simulink model "TxSteering_RxMVDR_4x4_HDL_IQ"  (R2023a)
settings: Solver=FixedStepDiscrete  StartTime=0.0  StopTime=stoptime  RelTol=1e-3
PreLoadFcn:
  | model_init
InitFcn:
  | model_init
model workspace (MAT data in the model file):
  socvcb = containers.Map
  socvcb.serialization.keys = {}
  socvcb.serialization.values = {}
  socvcb.serialization.uniformity = 0
  socvcb.serialization.keyType = 'double'
  socvcb.serialization.valueType = 'any'
values from neighbouring files (symbols this model uses):
  diagLoading = 5e-3    (= 0.005)    [model_init.m]
  dmaFIFOLength = 2^nextpow2(testSrc1.FrameLength*testSrc1.SamplesPerSymbol*2)    [model_init.m]
  fc = ConverterSampleRate*7/16    (= 860160000)    [model_init.m]
  FPGAClkRate = DataSampleRate/VectorSamplingFactor    (= 245760000)    [model_init.m]
  movavg_bitshift = nextpow2(windowSize)    [model_init.m]
  mvdrPipelineDelay = covMatDelay+movAvgDelay+matrixSolveDelay+normResponseDelay    [model_init.m]
  NCO_bits = 14    [model_init.m]
  numArrayElements = 4    [model_init.m]
  NumChan = 4    [model_init.m]
  reciprocalDelay = nextpow2(reciprocalin_dt.WordLength) + 1 + reciprocalin_dt.WordLength + 2      - strcmp(reciprocalin_dt.Signedness,'Signed') + 7    [model_init.m]
  rx_mag_delay = input_dt.WordLength + 2 + ceil(log2(NumChan)) + 1 + rx_mag_window_size    [model_init.m]
  rx_mag_inverse_delay = nextpow2(rx_mag_dt.WordLength) + 1 + rx_mag_dt.WordLength + 2 + 7    [model_init.m]
  rx_mag_sum_growth = nextpow2(rx_mag_window_size)    [model_init.m]
  rx_mag_window_size = 256    [model_init.m]
  s2mmFrameSize = testSrc1.FrameLength*testSrc1.SamplesPerSymbol*3    [model_init.m]
  testSrc1 = struct()    [model_init.m]
  testSrc2 = struct()    [model_init.m]
  windowSize = 4096    [model_init.m]
undefined symbols (not defined in the file or in its folder): Add, j, NumBits1, NumBits2, physconst, Shift
libraries: hdlsllib x29, simulink x15, embreciprocals x2, dspsrcs4 x2, dsphdlmathfun2 x1, embsystolicmatrixops x1, dsphdlsigops2 x1, commrfcorlib x1
(part 1 of 3)
Description:
  | MVDR RFSoC example for ZCU111
  | 
  | Copyright 2021 The MathWorks, Inc.
settings Model: DataTypeOverride=Off  SimulationMode=accelerator  Creator=mfornero  LastModifiedBy=tmealey
settings SolverCC: AlgebraicLoopSolver=TrustRegion
settings DataIOCC: SaveOutput=off  SaveTime=off
settings OptimizationCC: BlockReduction=off  ConditionallyExecuteInputs=off  DefaultParameterBehavior=Inlined  ReuseModelBlockBuffer=off  LifeSpan=inf
settings DebuggingCC: AlgebraicLoopMsg=error  SingleTaskRateTransMsg=error  ParameterPrecisionLossMsg=none  UnconnectedInputMsg=warning  UnconnectedOutputMsg=warning  UnconnectedLineMsg=warning  PregeneratedLibrarySubsystemCodeDiagnostic=none  StrictBusMsg=ErrorOnBusTreatedAsVector  SFUnexpectedBacktrackingDiag=warning  SFNoUnconditionalDefaultTransitionDiag=warning  SFExecutionAtInitializationDiag=none  ArithmeticOperatorsInVariantConditions=warning
settings HardwareCC: ProdBitPerPointer=32  ProdBitPerSizeT=32  ProdBitPerPtrDiffT=32  ProdLargestAtomicFloat=None  ProdIntDivRoundTo=Undefined  ProdEndianess=Unspecified  ProdWordSize=32  ProdHWDeviceType=ASIC/FPGA->ASIC/FPGA  ProdEqTarget=off
settings ModelReferenceCC: EnableRefExpFcnMdlSchedulingChecks=on
settings SFSimCC: SimUseLocalCustomCode=off  CustomCodeUndefinedFunction=UseInterfaceOnly
settings RTWCC: RTWUseLocalCustomCode=off  DLArmComputeVersion=19.05
settings CodeAppCC: StateflowObjectComments=on
settings GRTTargetCC: TargetLangStandard=C89/C90 (ANSI)
settings ConfigComp: CovMetricSettings=dw  CovSaveCumulativeToWorkspaceVar=on  CovSaveSingleToWorkspaceVar=on  CovExternalEMLEnable=off

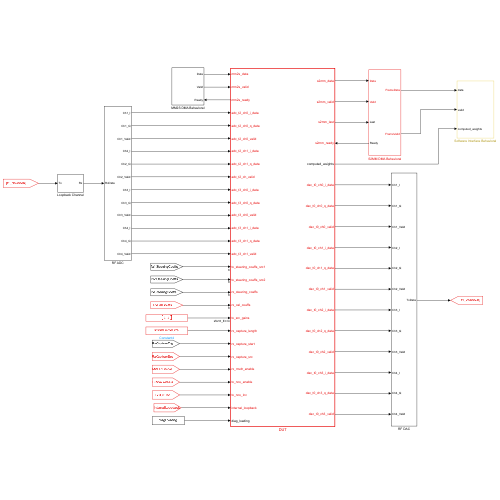
[thumbnail: Simulink's stored preview of the top-level diagram]
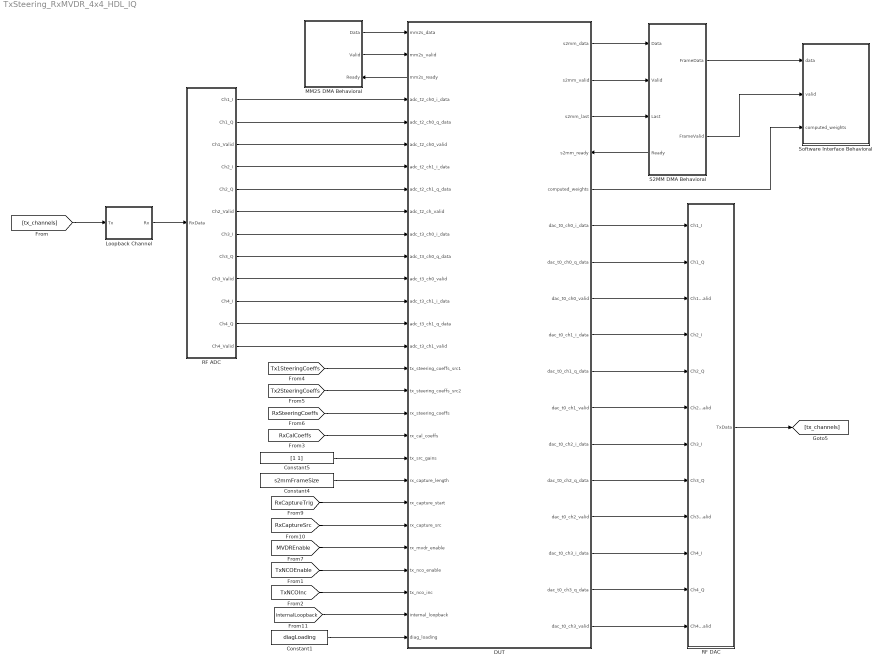
== system TxSteering_RxMVDR_4x4_HDL_IQ ==
  Constant1 : Constant  Value=diagLoading  OutDataTypeStr=matrixdivin_dt  SampleTime=-1
  Constant4 : Constant  Value=s2mmFrameSize  OutDataTypeStr=uint32  SampleTime=-1
  Constant5 : Constant  Value=[1 1]  OutDataTypeStr=tx_gain_dt  SampleTime=-1
  DUT : Subsystem  TreatAsAtomicUnit=on
      settings: PortSchema="{\"entries\":[{\"content\":{\"sides\":[{\"content\":{\"connectorIds\":[\"In1\",\"In2\",\"Out17\",\"In3\",\"In4\",\"In5\",\"In6\",\"In7\",\"In8\",\"In9\",\"In10\",\"In11\",\"In12\",\"In13\",\"In14\",\"In15\",\"In16\",\"In17\",\"In18\",\"In19\",\"In20\",\"In21\",\"In22\",\"In23\",\"In24\",\"In25\",\"In26\",\"In27\"]},\"type\":\"ConnectorPlacement.EquallySpacedRectSide\",\"uuid\":\"5cbbc5c1-13a2-4dd5-b798-0d6aa5a3512c\"},{\"content\":{\"connectorIds\":[\"Out1\",\"Out2\",\"Out3\",\"In28\",\"Out4\",\"Out5\",\"Out6\",\"Out7\",\"Out8\",\"Out9\",\"Out10\",\"Out11\",\"Out12\",\"Out13\",\"Out14\",\"Out15\",\"Out16\"],\"side\":\"RIGHT\"},\"type\":\"ConnectorPlacement.EquallySpacedRectSide\",\"uuid\":\"078c6bc6-159b-4e6a-9020-aaf50b1c87f6\"},{\"content\":{\"side\":\"TOP\"},\"type\":\"ConnectorPlacement.EquallySpacedRectSide\",\"uuid\":\"5dec20bf-c028-4555-acb0-00d4e0bd1eb1\"},{\"content\":{\"side\":\"HIDDEN\"},\"type\":\"ConnectorPlacement.EquallySpacedRectSide\",\"uuid\":\"f104c99f-3c00-46d1-a3ab-da9a095ae20c\"}]},\"type\":\"ConnectorPlacement.EquallySpacedConnector\",\"uuid\":\"99ff154b-6e8c-428f-8f67-53aff3cd9053\"}],\"packageUris\":[\"http://schema.mathworks.com/mf0/Connector/R2020b\"],\"version\":\"1.0\"}"
  Loopback Channel : Subsystem
  MM2S DMA Behavioral : Subsystem
      settings: PortSchema="{\"entries\":[{\"content\":{\"sides\":[{\"content\":{\"connectorIds\":[]},\"type\":\"ConnectorPlacement.EquallySpacedRectSide\",\"uuid\":\"6e5a1ec8-43bd-4e5c-bb67-adc7e52f765e\"},{\"content\":{\"connectorIds\":[\"Out1\",\"Out2\",\"In1\"],\"side\":\"RIGHT\"},\"type\":\"ConnectorPlacement.EquallySpacedRectSide\",\"uuid\":\"3e14b147-97a5-457d-828e-9dc648279d0e\"},{\"content\":{\"connectorIds\":[],\"side\":\"TOP\"},\"type\":\"ConnectorPlacement.EquallySpacedRectSide\",\"uuid\":\"b499ca48-b31e-4779-aede-04dca658d330\"},{\"content\":{\"connectorIds\":[],\"side\":\"HIDDEN\"},\"type\":\"ConnectorPlacement.EquallySpacedRectSide\",\"uuid\":\"e46e2562-9ab1-42db-980c-487b803af873\"}]},\"type\":\"ConnectorPlacement.EquallySpacedConnector\",\"uuid\":\"234057b8-4ead-4b5a-9893-76ff1204f271\"}],\"packageUris\":[\"http://schema.mathworks.com/mf0/Connector/R2020b\"],\"version\":\"1.0\"}"
  RF ADC : Subsystem
  RF DAC : Subsystem
  S2MM DMA Behavioral : Subsystem
      settings: PortSchema="{\"entries\":[{\"content\":{\"sides\":[{\"content\":{\"connectorIds\":[\"In1\",\"In2\",\"In3\",\"Out3\"]},\"type\":\"ConnectorPlacement.EquallySpacedRectSide\",\"uuid\":\"f5aebce5-d24c-432e-8d9d-6ae810fc0a64\"},{\"content\":{\"connectorIds\":[\"Out1\",\"Out2\"],\"side\":\"RIGHT\"},\"type\":\"ConnectorPlacement.EquallySpacedRectSide\",\"uuid\":\"87d7b61c-1b18-489c-87d0-263bc891b967\"},{\"content\":{\"side\":\"TOP\"},\"type\":\"ConnectorPlacement.EquallySpacedRectSide\",\"uuid\":\"c0471b66-642d-47c1-93a8-85d0262e809a\"},{\"content\":{\"side\":\"HIDDEN\"},\"type\":\"ConnectorPlacement.EquallySpacedRectSide\",\"uuid\":\"468d2625-6b9b-4b39-93eb-7f122a4e72a5\"}]},\"type\":\"ConnectorPlacement.EquallySpacedConnector\",\"uuid\":\"6af60fba-ab37-47d2-9d8a-dd48226214e6\"}],\"packageUris\":[\"http://schema.mathworks.com/mf0/Connector/R2020b\"],\"version\":\"1.0\"}"
  Software Interface Behavioral : Subsystem
  wires:
  [InternalLoopback] -> DUT/26(internal_loopback)
  Constant5/1 -> DUT/19(tx_src_gains)
  Constant4/1 -> DUT/20(rx_capture_length)
  [RxCaptureTrig] -> DUT/21(rx_capture_start)
  [RxCaptureSrc] -> DUT/22(rx_capture_src)
  DUT/5(dac_t0_ch0_i_data) -> RF DAC/1(Ch1_I)
  DUT/6(dac_t0_ch0_q_data) -> RF DAC/2(Ch1_Q)
  DUT/7(dac_t0_ch0_valid) -> RF DAC/3(Ch1_Valid)
  DUT/8(dac_t0_ch1_i_data) -> RF DAC/4(Ch2_I)
  DUT/9(dac_t0_ch1_q_data) -> RF DAC/5(Ch2_Q)
  DUT/10(dac_t0_ch1_valid) -> RF DAC/6(Ch2_Valid)
  DUT/11(dac_t0_ch2_i_data) -> RF DAC/7(Ch3_I)
  DUT/12(dac_t0_ch2_q_data) -> RF DAC/8(Ch3_Q)
  DUT/13(dac_t0_ch2_valid) -> RF DAC/9(Ch3_Valid)
  DUT/14(dac_t0_ch3_i_data) -> RF DAC/10(Ch4_I)
  DUT/15(dac_t0_ch3_q_data) -> RF DAC/11(Ch4_Q)
  DUT/16(dac_t0_ch3_valid) -> RF DAC/12(Ch4_Valid)
  RF DAC/1(TxData) -> [tx_channels]
  [tx_channels] -> Loopback Channel/1(Tx)
  Loopback Channel/1(Rx) -> RF ADC/1(RxData)
  [TxNCOEnable] -> DUT/24(tx_nco_enable)
  [TxNCOInc] -> DUT/25(tx_nco_inc)
  S2MM DMA Behavioral/3(Ready) -> DUT/28(s2mm_ready)
  S2MM DMA Behavioral/1(FrameData) -> Software Interface Behavioral/1(data)
  S2MM DMA Behavioral/2(FrameValid) -> Software Interface Behavioral/2(valid)
  DUT/4(computed_weights) -> Software Interface Behavioral/3(computed_weights)
  DUT/1(s2mm_data) -> S2MM DMA Behavioral/1(Data)
  DUT/2(s2mm_valid) -> S2MM DMA Behavioral/2(Valid)
  MM2S DMA Behavioral/1(Data) -> DUT/1(mm2s_data)
  MM2S DMA Behavioral/2(Valid) -> DUT/2(mm2s_valid)
  DUT/17(mm2s_ready) -> MM2S DMA Behavioral/1(Ready)
  RF ADC/6(Ch2_Valid) -> DUT/8(adc_t2_ch_valid)
  RF ADC/7(Ch3_I) -> DUT/9(adc_t3_ch0_i_data)
  RF ADC/8(Ch3_Q) -> DUT/10(adc_t3_ch0_q_data)
  RF ADC/9(Ch3_Valid) -> DUT/11(adc_t3_ch0_valid)
  RF ADC/10(Ch4_I) -> DUT/12(adc_t3_ch1_i_data)
  RF ADC/11(Ch4_Q) -> DUT/13(adc_t3_ch1_q_data)
  RF ADC/12(Ch4_Valid) -> DUT/14(adc_t3_ch1_valid)
  [Tx1SteeringCoeffs] -> DUT/15(tx_steering_coeffs_src1)
  [Tx2SteeringCoeffs] -> DUT/16(tx_steering_coeffs_src2)
  [RxSteeringCoeffs] -> DUT/17(rx_steering_coeffs)
  [RxCalCoeffs] -> DUT/18(rx_cal_coeffs)
  DUT/3(s2mm_last) -> S2MM DMA Behavioral/3(Last)
  [MVDREnable] -> DUT/23(rx_mvdr_enable)
  RF ADC/1(Ch1_I) -> DUT/3(adc_t2_ch0_i_data)
  RF ADC/2(Ch1_Q) -> DUT/4(adc_t2_ch0_q_data)
  RF ADC/3(Ch1_Valid) -> DUT/5(adc_t2_ch0_valid)
  RF ADC/4(Ch2_I) -> DUT/6(adc_t2_ch1_i_data)
  RF ADC/5(Ch2_Q) -> DUT/7(adc_t2_ch1_q_data)
  Constant1/1 -> DUT/27(diag_loading)

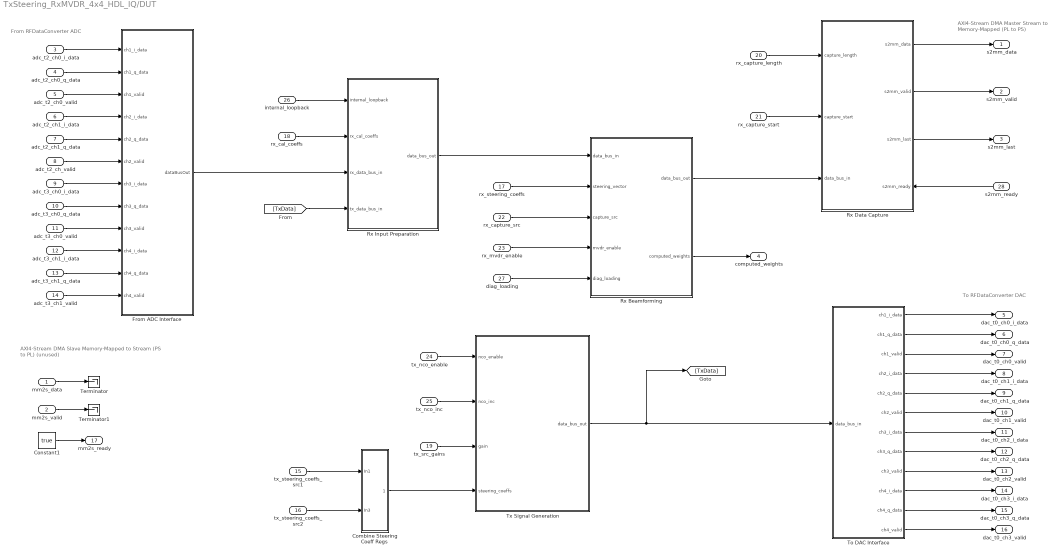
== system TxSteering_RxMVDR_4x4_HDL_IQ/DUT ==
  note: AXI4-Stream DMA Master
      | Stream to Memory-Mapped (PL to PS)
  note: AXI4-Stream DMA Slave
      | Memory-Mapped to Stream (PS to PL)
      | (unused)
  note: From RFDataConverter ADC
  note: To RFDataConverter DAC
  mm2s_data : Inport
  mm2s_valid : Inport  Port=2
  adc_t2_ch0_i_data : Inport  Port=3
  adc_t2_ch0_q_data : Inport  Port=4
  adc_t2_ch0_valid : Inport  Port=5
  adc_t2_ch1_i_data : Inport  Port=6
  adc_t2_ch1_q_data : Inport  Port=7
  adc_t2_ch_valid : Inport  Port=8
  adc_t3_ch0_i_data : Inport  Port=9
  adc_t3_ch0_q_data : Inport  Port=10
  adc_t3_ch0_valid : Inport  Port=11
  adc_t3_ch1_i_data : Inport  Port=12
  adc_t3_ch1_q_data : Inport  Port=13
  adc_t3_ch1_valid : Inport  Port=14
  tx_steering_coeffs_src1 : Inport  Port=15  PortDimensions=NumChan*2
  tx_steering_coeffs_src2 : Inport  Port=16  PortDimensions=NumChan*2
  rx_steering_coeffs : Inport  Port=17  PortDimensions=NumChan*2
  rx_cal_coeffs : Inport  Port=18  PortDimensions=NumChan*2
  tx_src_gains : Inport  Port=19  OutDataTypeStr=tx_gain_dt
  rx_capture_length : Inport  Port=20
  rx_capture_start : Inport  Port=21
  rx_capture_src : Inport  Port=22
  rx_mvdr_enable : Inport  Port=23
  tx_nco_enable : Inport  Port=24
  tx_nco_inc : Inport  Port=25
  internal_loopback : Inport  Port=26
  diag_loading : Inport  Port=27
  s2mm_ready : Inport  Port=28
  Combine Steering Coeff Regs : Subsystem
  Constant1 : Constant  Value=true  OutDataTypeStr=boolean  SampleTime=-1
  From ADC Interface : Subsystem
  Rx Beamforming : Subsystem
  Rx Data Capture : Subsystem
      settings: PortSchema="{\"entries\":[{\"content\":{\"sides\":[{\"content\":{\"connectorIds\":[\"In1\",\"In2\",\"In3\"]},\"type\":\"ConnectorPlacement.EquallySpacedRectSide\",\"uuid\":\"3ce440ad-60a3-40a1-9abc-8b07e8479e74\"},{\"content\":{\"connectorIds\":[\"Out1\",\"Out2\",\"Out3\",\"In4\"],\"side\":\"RIGHT\"},\"type\":\"ConnectorPlacement.EquallySpacedRectSide\",\"uuid\":\"92cb9a6e-31c8-4c68-811d-5cb9de201228\"},{\"content\":{\"side\":\"TOP\"},\"type\":\"ConnectorPlacement.EquallySpacedRectSide\",\"uuid\":\"4ff664a1-3d68-43c3-89c1-825c045b6984\"},{\"content\":{\"side\":\"HIDDEN\"},\"type\":\"ConnectorPlacement.EquallySpacedRectSide\",\"uuid\":\"ea40c324-81e0-4145-89f3-1e0de81d6070\"}]},\"type\":\"ConnectorPlacement.EquallySpacedConnector\",\"uuid\":\"89aac716-5ee7-4b56-a06e-6874cb9890cb\"}],\"packageUris\":[\"http://schema.mathworks.com/mf0/Connector/R2020b\"],\"version\":\"1.0\"}"
  Rx Input Preparation : Subsystem
  Terminator : Terminator
  Terminator1 : Terminator
  To DAC Interface : Subsystem
  Tx Signal Generation : Subsystem
  s2mm_data : Outport  VectorParamsAs1DForOutWhenUnconnected=off
  s2mm_valid : Outport  Port=2  VectorParamsAs1DForOutWhenUnconnected=off
  s2mm_last : Outport  Port=3  VectorParamsAs1DForOutWhenUnconnected=off
  computed_weights : Outport  Port=4
  dac_t0_ch0_i_data : Outport  Port=5  VectorParamsAs1DForOutWhenUnconnected=off
  dac_t0_ch0_q_data : Outport  Port=6  VectorParamsAs1DForOutWhenUnconnected=off
  dac_t0_ch0_valid : Outport  Port=7  VectorParamsAs1DForOutWhenUnconnected=off
  dac_t0_ch1_i_data : Outport  Port=8  VectorParamsAs1DForOutWhenUnconnected=off
  dac_t0_ch1_q_data : Outport  Port=9  VectorParamsAs1DForOutWhenUnconnected=off
  dac_t0_ch1_valid : Outport  Port=10  VectorParamsAs1DForOutWhenUnconnected=off
  dac_t0_ch2_i_data : Outport  Port=11  VectorParamsAs1DForOutWhenUnconnected=off
  dac_t0_ch2_q_data : Outport  Port=12  VectorParamsAs1DForOutWhenUnconnected=off
  dac_t0_ch2_valid : Outport  Port=13  VectorParamsAs1DForOutWhenUnconnected=off
  dac_t0_ch3_i_data : Outport  Port=14  VectorParamsAs1DForOutWhenUnconnected=off
  dac_t0_ch3_q_data : Outport  Port=15  VectorParamsAs1DForOutWhenUnconnected=off
  dac_t0_ch3_valid : Outport  Port=16  VectorParamsAs1DForOutWhenUnconnected=off
  mm2s_ready : Outport  Port=17  VectorParamsAs1DForOutWhenUnconnected=off
  wires:
  Constant1/1 -> mm2s_ready/1
  s2mm_ready/1 -> Rx Data Capture/4(s2mm_ready)
  rx_capture_length/1 -> Rx Data Capture/1(capture_length)
  rx_capture_start/1 -> Rx Data Capture/2(capture_start)
  Rx Data Capture/2(s2mm_valid) -> s2mm_valid/1
  Rx Data Capture/1(s2mm_data) -> s2mm_data/1
  adc_t2_ch0_i_data/1 -> From ADC Interface/1("ch1_i_data ")
  adc_t2_ch0_valid/1 -> From ADC Interface/3(ch1_valid)
  adc_t2_ch0_q_data/1 -> From ADC Interface/2(ch1_q_data)
  adc_t2_ch1_i_data/1 -> From ADC Interface/4(ch2_i_data)
  adc_t2_ch_valid/1 -> From ADC Interface/6(ch2_valid)
  adc_t2_ch1_q_data/1 -> From ADC Interface/5(ch2_q_data)
  adc_t3_ch0_i_data/1 -> From ADC Interface/7(ch3_i_data)
  adc_t3_ch0_valid/1 -> From ADC Interface/9(ch3_valid)
  adc_t3_ch0_q_data/1 -> From ADC Interface/8(ch3_q_data)
  adc_t3_ch1_i_data/1 -> From ADC Interface/10(ch4_i_data)
  adc_t3_ch1_valid/1 -> From ADC Interface/12(ch4_valid)
  adc_t3_ch1_q_data/1 -> From ADC Interface/11(ch4_q_data)
  mm2s_data/1 -> Terminator/1
  mm2s_valid/1 -> Terminator1/1
  To DAC Interface/1(ch1_i_data) -> dac_t0_ch0_i_data/1
  To DAC Interface/2(ch1_q_data) -> dac_t0_ch0_q_data/1
  To DAC Interface/3(ch1_valid) -> dac_t0_ch0_valid/1
  To DAC Interface/4(ch2_i_data) -> dac_t0_ch1_i_data/1
  To DAC Interface/5(ch2_q_data) -> dac_t0_ch1_q_data/1
  To DAC Interface/6(ch2_valid) -> dac_t0_ch1_valid/1
  To DAC Interface/7(ch3_i_data) -> dac_t0_ch2_i_data/1
  To DAC Interface/8(ch3_q_data) -> dac_t0_ch2_q_data/1
  To DAC Interface/9(ch3_valid) -> dac_t0_ch2_valid/1
  To DAC Interface/10(ch4_i_data) -> dac_t0_ch3_i_data/1
  To DAC Interface/11(ch4_q_data) -> dac_t0_ch3_q_data/1
  To DAC Interface/12(ch4_valid) -> dac_t0_ch3_valid/1
  rx_steering_coeffs/1 -> Rx Beamforming/2(steering_vector)
  tx_steering_coeffs_src1/1 -> Combine Steering Coeff Regs/1(In1)
  tx_steering_coeffs_src2/1 -> Combine Steering Coeff Regs/2(In3)
  [TxData] -> Rx Input Preparation/4(tx_data_bus_in)
  rx_capture_src/1 -> Rx Beamforming/3(capture_src)
  internal_loopback/1 -> Rx Input Preparation/1(internal_loopback)
  rx_cal_coeffs/1 -> Rx Input Preparation/2(rx_cal_coeffs)
  Tx Signal Generation/1(data_bus_out) -> [TxData], To DAC Interface/1(data_bus_in)
  Combine Steering Coeff Regs/1(Out1) -> Tx Signal Generation/4(steering_coeffs)
  tx_src_gains/1 -> Tx Signal Generation/3(gain)
  Rx Input Preparation/1(data_bus_out) -> Rx Beamforming/1(data_bus_in)
  From ADC Interface/1(dataBusOut) -> Rx Input Preparation/3(rx_data_bus_in)
  tx_nco_inc/1 -> Tx Signal Generation/2(nco_inc)
  tx_nco_enable/1 -> Tx Signal Generation/1(nco_enable)
  Rx Beamforming/2(computed_weights) -> computed_weights/1
  Rx Beamforming/1(data_bus_out) -> Rx Data Capture/3(data_bus_in)
  Rx Data Capture/3(s2mm_last) -> s2mm_last/1
  rx_mvdr_enable/1 -> Rx Beamforming/4(mvdr_enable)
  diag_loading/1 -> Rx Beamforming/5(diag_loading)

== system TxSteering_RxMVDR_4x4_HDL_IQ/Loopback Channel ==
  Tx : Inport
  Apply Channel Noise : Subsystem
  Apply Phase/Amplitude imbalance : Subsystem
  Delay1 : Delay  DelayLength=1
  Gain : Gain  Gain=0.15
  Rx : Outport
  wires:
  Tx/1 -> Delay1/1
  Delay1/1 -> Gain/1
  Apply Phase/Amplitude imbalance/1(Out1) -> Apply Channel Noise/1(In1)
  Apply Channel Noise/1(Rx) -> Rx/1
  Gain/1 -> Apply Phase/Amplitude imbalance/1(In1)

== system TxSteering_RxMVDR_4x4_HDL_IQ/MM2S DMA Behavioral ==
  Ready : Inport
  Constant6 : Constant  Value=false  SampleTime=-1
  Constant7 : Constant  Value=0  OutDataTypeStr=fixdt(0,128,0)  SampleTime=-1
  Terminator : Terminator
  Data : Outport
  Valid : Outport  Port=2
  wires:
  Constant7/1 -> Data/1
  Constant6/1 -> Valid/1
  Ready/1 -> Terminator/1

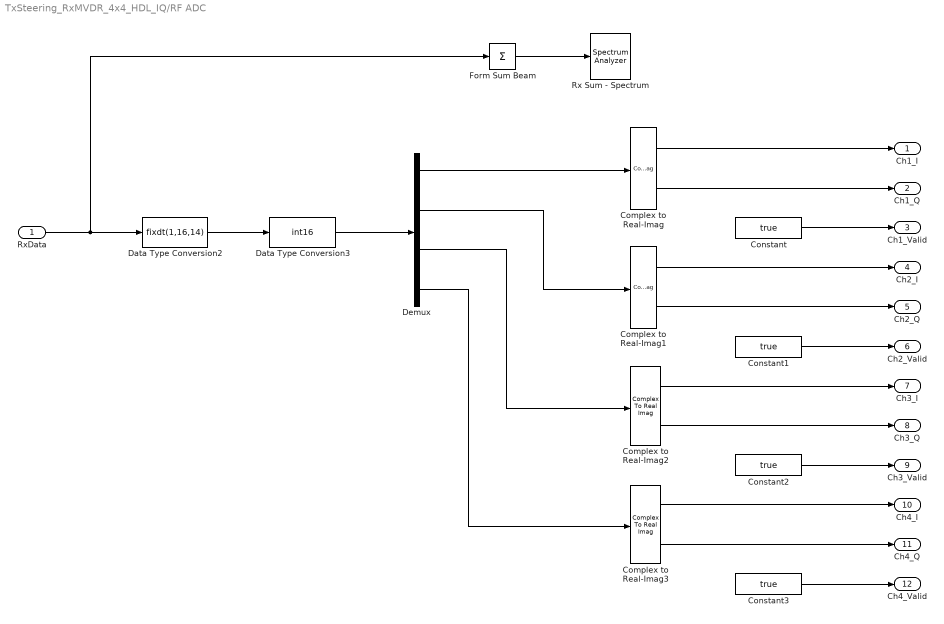
== system TxSteering_RxMVDR_4x4_HDL_IQ/RF ADC ==
  RxData : Inport
  Complex to Real-Imag{,1..3} (4 alike) : ComplexToRealImag
  Constant{,1..3} (4 alike) : Constant  Value=true  SampleTime=-1
  Data Type Conversion2 : DataTypeConversion  OutDataTypeStr=fixdt(1,16,14)  SaturateOnIntegerOverflow=off  RndMeth=Floor
  Data Type Conversion3 : DataTypeConversion  OutDataTypeStr=int16  ConvertRealWorld=Stored Integer (SI)  SaturateOnIntegerOverflow=off  RndMeth=Floor
  Demux : Demux
  Form Sum Beam : Sum  Inputs=+
  Rx Sum - Spectrum : SpectrumAnalyzer  WindowPosition=[121.000000,133.000000,676.000000,509.000000,]  ScopeFrameLocation=window  Method=Welch  SampleRateSource=Property  SampleRate=DataSampleRate  Span=245760000  StartFrequency=-122880000  StopFrequency=122880000  AveragingMethod=Running  YLimits=[-95.95739742,7.93018941]
      settings: OpenAtSimulationStart=off
  Ch1_I : Outport
  Ch1_Q : Outport  Port=2
  Ch1_Valid : Outport  Port=3
  Ch2_I : Outport  Port=4
  Ch2_Q : Outport  Port=5
  Ch2_Valid : Outport  Port=6
  Ch3_I : Outport  Port=7
  Ch3_Q : Outport  Port=8
  Ch3_Valid : Outport  Port=9
  Ch4_I : Outport  Port=10
  Ch4_Q : Outport  Port=11
  Ch4_Valid : Outport  Port=12
  wires:
  Demux/4 -> Complex to Real-Imag3/1
  Complex to Real-Imag1/1 -> Ch2_I/1
  Demux/2 -> Complex to Real-Imag1/1
  Complex to Real-Imag2/2 -> Ch3_Q/1
  Complex to Real-Imag3/1 -> Ch4_I/1
  Demux/3 -> Complex to Real-Imag2/1
  Complex to Real-Imag2/1 -> Ch3_I/1
  Complex to Real-Imag3/2 -> Ch4_Q/1
  Complex to Real-Imag/2 -> Ch1_Q/1
  Complex to Real-Imag/1 -> Ch1_I/1
  Complex to Real-Imag1/2 -> Ch2_Q/1
  Constant/1 -> Ch1_Valid/1
  Demux/1 -> Complex to Real-Imag/1
  Constant1/1 -> Ch2_Valid/1
  Constant2/1 -> Ch3_Valid/1
  Constant3/1 -> Ch4_Valid/1
  Form Sum Beam/1 -> Rx Sum - Spectrum/1
  Data Type Conversion2/1 -> Data Type Conversion3/1
  Data Type Conversion3/1 -> Demux/1
  RxData/1 -> Form Sum Beam/1, Data Type Conversion2/1

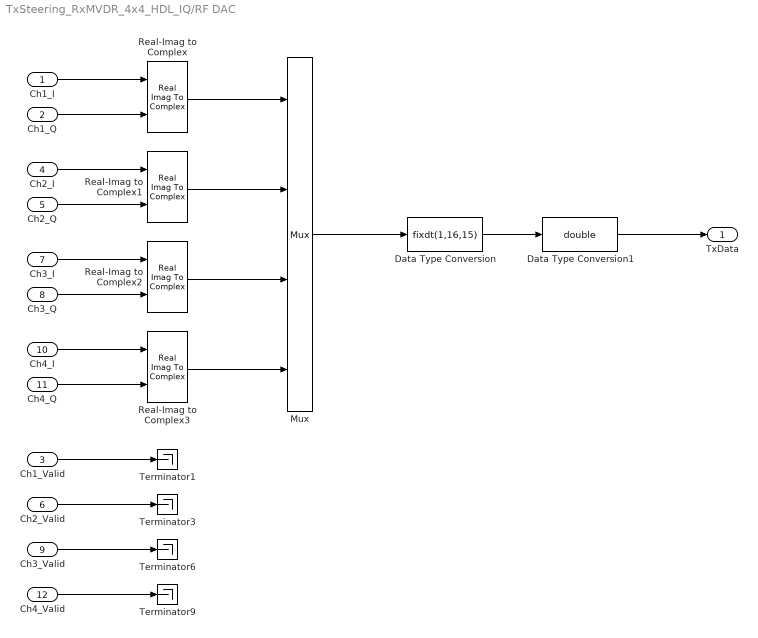
== system TxSteering_RxMVDR_4x4_HDL_IQ/RF DAC ==
  Ch1_I : Inport
  Ch1_Q : Inport  Port=2
  Ch1_Valid : Inport  Port=3
  Ch2_I : Inport  Port=4
  Ch2_Q : Inport  Port=5
  Ch2_Valid : Inport  Port=6
  Ch3_I : Inport  Port=7
  Ch3_Q : Inport  Port=8
  Ch3_Valid : Inport  Port=9
  Ch4_I : Inport  Port=10
  Ch4_Q : Inport  Port=11
  Ch4_Valid : Inport  Port=12
  Data Type Conversion : DataTypeConversion  OutDataTypeStr=fixdt(1,16,15)  ConvertRealWorld=Stored Integer (SI)  SaturateOnIntegerOverflow=off  RndMeth=Floor
  Data Type Conversion1 : DataTypeConversion  OutDataTypeStr=double  SaturateOnIntegerOverflow=off  RndMeth=Floor
  Mux : Mux
  Real-Imag to Complex{,1..3} (4 alike) : RealImagToComplex
  Terminator{1,3,6,9} (4 alike) : Terminator
  TxData : Outport
  wires:
  Ch2_Q/1 -> Real-Imag to Complex1/2
  Ch2_Valid/1 -> Terminator3/1
  Ch3_Valid/1 -> Terminator6/1
  Ch1_Valid/1 -> Terminator1/1
  Ch4_I/1 -> Real-Imag to Complex3/1
  Ch4_Q/1 -> Real-Imag to Complex3/2
  Ch3_Q/1 -> Real-Imag to Complex2/2
  Ch4_Valid/1 -> Terminator9/1
  Ch1_Q/1 -> Real-Imag to Complex/2
  Ch1_I/1 -> Real-Imag to Complex/1
  Ch2_I/1 -> Real-Imag to Complex1/1
  Ch3_I/1 -> Real-Imag to Complex2/1
  Real-Imag to Complex/1 -> Mux/1
  Real-Imag to Complex1/1 -> Mux/2
  Real-Imag to Complex2/1 -> Mux/3
  Real-Imag to Complex3/1 -> Mux/4
  Data Type Conversion/1 -> Data Type Conversion1/1
  Mux/1 -> Data Type Conversion/1
  Data Type Conversion1/1 -> TxData/1

== system TxSteering_RxMVDR_4x4_HDL_IQ/S2MM DMA Behavioral ==
  Data : Inport
  Valid : Inport  Port=2
  Last : Inport  Port=3
  AXI Stream Deserializer : MATLAB Function  TreatAsAtomicUnit=on  mask{FRAME_SIZE=s2mmFrameSize}
      mask prompts: FRAME_SIZE "Frame size:"
  Constant10 : Constant  Value=true  SampleTime=-1
  Delay : Delay  DelayLength=1
  Delay1 : Delay  DelayLength=1
  To Workspace : ToWorkspace  VariableName=sim_dma_valid  SampleTime=-1
      settings: Save2DSignal=2-D array (concatenate along first dimension)
  To Workspace1 : ToWorkspace  VariableName=sim_dma_last  SampleTime=-1
      settings: Save2DSignal=2-D array (concatenate along first dimension)
  To Workspace2 : ToWorkspace  VariableName=sim_dma_data  SampleTime=-1
      settings: Save2DSignal=2-D array (concatenate along first dimension)
  Unpack to uint32 : Subsystem
  FrameData : Outport
  FrameValid : Outport  Port=2
  Ready : Outport  Port=3
  wires:
  Data/1 -> To Workspace2/1, AXI Stream Deserializer/1(data_i)
  Valid/1 -> To Workspace/1, AXI Stream Deserializer/2(valid_i)
  Constant10/1 -> Ready/1
  AXI Stream Deserializer/1(data_o) -> Delay/1
  AXI Stream Deserializer/2(valid_o) -> Delay1/1
  Unpack to uint32/1(dataOut) -> FrameData/1
  Unpack to uint32/2(validOut) -> FrameValid/1
  Delay/1 -> Unpack to uint32/1(dataIn)
  Delay1/1 -> Unpack to uint32/2(validIn)
  Last/1 -> To Workspace1/1

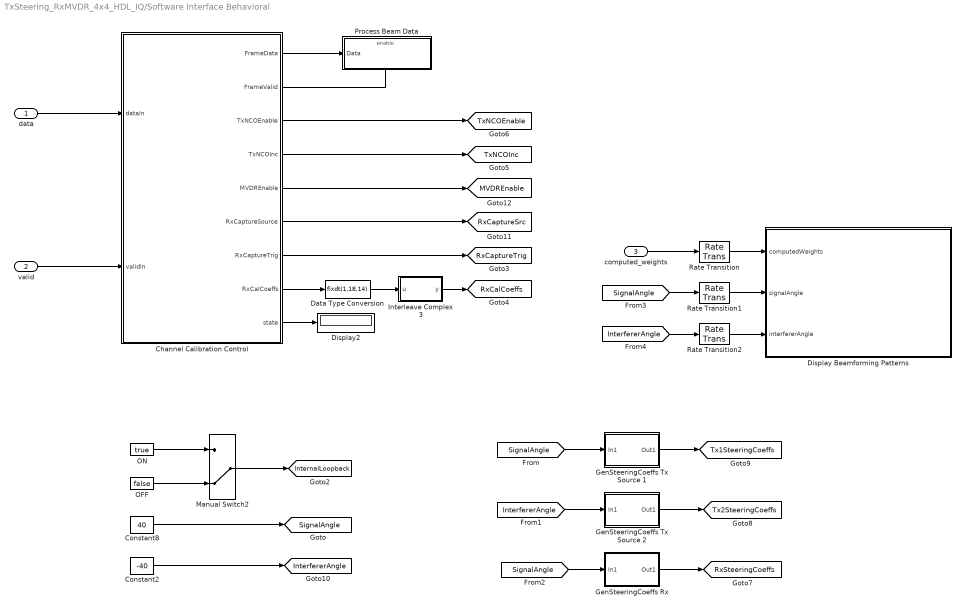
== system TxSteering_RxMVDR_4x4_HDL_IQ/Software Interface Behavioral ==
  data : Inport
  valid : Inport  Port=2
  computed_weights : Inport  Port=3
  Channel Calibration Control : MATLAB Function  TreatAsAtomicUnit=on
      mask init:
      | % Suppress warning for overflow from reinterpretcast
      | Simulink.suppressDiagnostic(gcb,...
      |  'Stateflow:Runtime:DataOverflowErrorMSLD');
  Constant2 : Constant  Value=-40  OutDataTypeStr=double  SampleTime=-1
  Constant8 : Constant  Value=40  OutDataTypeStr=double  SampleTime=-1
  Data Type Conversion : DataTypeConversion  OutDataTypeStr=fixdt(1,18,14)  SaturateOnIntegerOverflow=off  RndMeth=Floor
  Display Beamforming Patterns : MATLAB Function  TreatAsAtomicUnit=on
  Display2 : Display
  GenSteeringCoeffs Rx : Subsystem
  GenSteeringCoeffs Tx Source 1 : Subsystem
  GenSteeringCoeffs Tx Source 2 : Subsystem
  Interleave Complex 3 : Subsystem  mask(Interleave Complex){}
      mask help: Interleave real and imaginary components. Output is a vector with twice the length of the input.
      mask Display: fprintf('Interleave\nComplex');
  Manual Switch2 : ManualSwitch  CurrentSetting=0
  OFF : Constant  Value=false  OutDataTypeStr=boolean  SampleTime=-1
  ON : Constant  Value=true  OutDataTypeStr=boolean  SampleTime=-1
  Process Beam Data : Subsystem
  Rate Transition : RateTransition  OutPortSampleTimeOpt=Multiple of input port sample time  OutPortSampleTimeMultiple=256
  Rate Transition1 : RateTransition  OutPortSampleTimeOpt=Multiple of input port sample time  OutPortSampleTimeMultiple=256
  Rate Transition2 : RateTransition  OutPortSampleTimeOpt=Multiple of input port sample time  OutPortSampleTimeMultiple=256
  tag scope: InterfererAngle=global, InternalLoopback=global, MVDREnable=global, RxCalCoeffs=global, RxCaptureSrc=global, RxCaptureTrig=global, RxSteeringCoeffs=global, SignalAngle=global, Tx1SteeringCoeffs=global, Tx2SteeringCoeffs=global, TxNCOEnable=global, TxNCOInc=global
  wires:
  Channel Calibration Control/5(MVDREnable) -> [MVDREnable]
  OFF/1 -> Manual Switch2/2
  Manual Switch2/1 -> [InternalLoopback]
  ON/1 -> Manual Switch2/1
  data/1 -> Channel Calibration Control/1(dataIn)
  valid/1 -> Channel Calibration Control/2(validIn)
  Channel Calibration Control/4(TxNCOInc) -> [TxNCOInc]
  Channel Calibration Control/3(TxNCOEnable) -> [TxNCOEnable]
  Channel Calibration Control/1(FrameData) -> Process Beam Data/1(Data)
  GenSteeringCoeffs Rx/1(Out1) -> [RxSteeringCoeffs]
  GenSteeringCoeffs Tx Source 2/1(Out1) -> [Tx2SteeringCoeffs]
  GenSteeringCoeffs Tx Source 1/1(Out1) -> [Tx1SteeringCoeffs]
  Constant8/1 -> [SignalAngle]
  Constant2/1 -> [InterfererAngle]
  [SignalAngle] -> GenSteeringCoeffs Tx Source 1/1(In1)
  [InterfererAngle] -> GenSteeringCoeffs Tx Source 2/1(In1)
  [SignalAngle] -> GenSteeringCoeffs Rx/1(In1)
  computed_weights/1 -> Rate Transition/1
  [SignalAngle] -> Rate Transition1/1
  [InterfererAngle] -> Rate Transition2/1
  Rate Transition/1 -> Display Beamforming Patterns/1(computedWeights)
  Rate Transition1/1 -> Display Beamforming Patterns/2(signalAngle)
  Rate Transition2/1 -> Display Beamforming Patterns/3(interfererAngle)
  Channel Calibration Control/2(FrameValid) -> Process Beam Data/Enable
  Data Type Conversion/1 -> Interleave Complex 3/1(u)
  Channel Calibration Control/8(RxCalCoeffs) -> Data Type Conversion/1
  Interleave Complex 3/1(y) -> [RxCalCoeffs]
  Channel Calibration Control/6(RxCaptureSource) -> [RxCaptureSrc]
  Channel Calibration Control/7(RxCaptureTrig) -> [RxCaptureTrig]
  Channel Calibration Control/9(state) -> Display2/1

== system TxSteering_RxMVDR_4x4_HDL_IQ/DUT/Combine Steering Coeff Regs ==
  In1 : Inport
  In3 : Inport  Port=2
  Deinterleave Complex : Subsystem  mask(Deinterleave Complex){}
      mask help: Deinterleave real and imaginary components from input vector. Output is a vector with half the length of the input.
      mask Display: fprintf('Deinterleave\nComplex');
  Deinterleave Complex1 : Subsystem  mask(Deinterleave Complex){}
      mask help: Deinterleave real and imaginary components from input vector. Output is a vector with half the length of the input.
      mask Display: fprintf('Deinterleave\nComplex');
  Vector Concatenate : Concatenate
  Out1 : Outport
  wires:
  Vector Concatenate/1 -> Out1/1
  Deinterleave Complex/1(y) -> Vector Concatenate/1
  In1/1 -> Deinterleave Complex/1(u)
  In3/1 -> Deinterleave Complex1/1(u)
  Deinterleave Complex1/1(y) -> Vector Concatenate/2

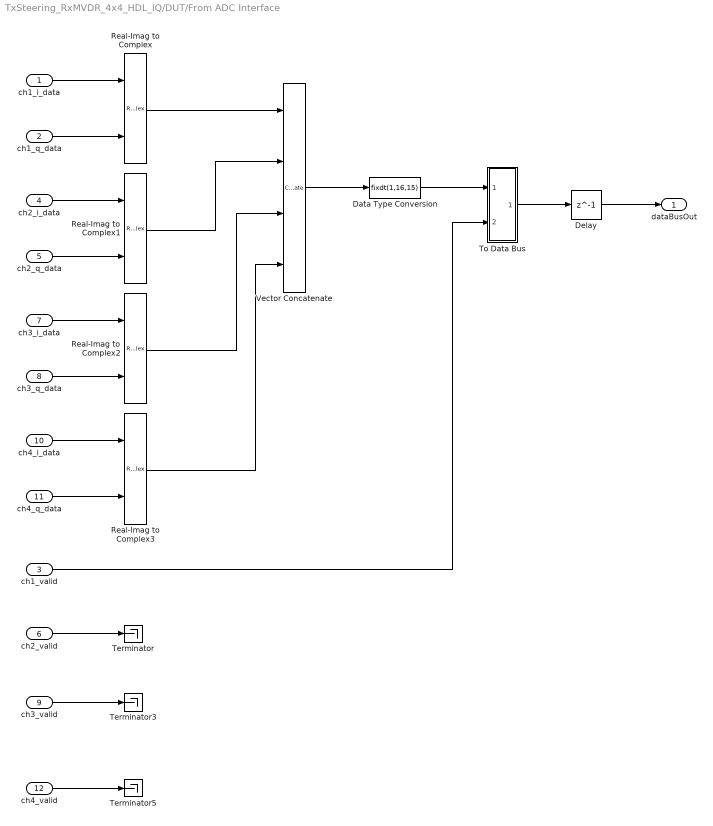
== system TxSteering_RxMVDR_4x4_HDL_IQ/DUT/From ADC Interface ==
  "ch1_i_data " : Inport
  ch1_q_data : Inport  Port=2
  ch1_valid : Inport  Port=3
  ch2_i_data : Inport  Port=4
  ch2_q_data : Inport  Port=5
  ch2_valid : Inport  Port=6
  ch3_i_data : Inport  Port=7
  ch3_q_data : Inport  Port=8
  ch3_valid : Inport  Port=9
  ch4_i_data : Inport  Port=10
  ch4_q_data : Inport  Port=11
  ch4_valid : Inport  Port=12
  Data Type Conversion : DataTypeConversion  OutDataTypeStr=fixdt(1,16,15)  ConvertRealWorld=Stored Integer (SI)  SaturateOnIntegerOverflow=off  RndMeth=Floor
  Delay : Delay  DelayLength=1
  Real-Imag to Complex{,1..3} (4 alike) : RealImagToComplex
  Terminator : Terminator
  Terminator3 : Terminator
  Terminator5 : Terminator
  To Data Bus : Subsystem  mask(To Data Bus){dummy=0}
      mask help: Create a streaming Data Bus from Data and Valid signals.
      mask Display:
      | port_label('input',1,'data');
      | port_label('input',2,'valid');
  Vector Concatenate : Concatenate  NumInputs=4  Mode=Multidimensional array  ConcatenateDimension=2
  dataBusOut : Outport  VectorParamsAs1DForOutWhenUnconnected=off
  wires:
  ch2_valid/1 -> Terminator/1
  ch3_valid/1 -> Terminator3/1
  ch4_valid/1 -> Terminator5/1
  Real-Imag to Complex/1 -> Vector Concatenate/1
  Real-Imag to Complex1/1 -> Vector Concatenate/2
  Real-Imag to Complex2/1 -> Vector Concatenate/3
  Real-Imag to Complex3/1 -> Vector Concatenate/4
  "ch1_i_data "/1 -> Real-Imag to Complex/1
  ch1_q_data/1 -> Real-Imag to Complex/2
  ch2_i_data/1 -> Real-Imag to Complex1/1
  ch2_q_data/1 -> Real-Imag to Complex1/2
  ch3_i_data/1 -> Real-Imag to Complex2/1
  ch3_q_data/1 -> Real-Imag to Complex2/2
  ch4_i_data/1 -> Real-Imag to Complex3/1
  ch4_q_data/1 -> Real-Imag to Complex3/2
  Vector Concatenate/1 -> Data Type Conversion/1
  ch1_valid/1 -> To Data Bus/2(valid)
  To Data Bus/1(bus) -> Delay/1
  Data Type Conversion/1 -> To Data Bus/1(data)
  Delay/1 -> dataBusOut/1

== system TxSteering_RxMVDR_4x4_HDL_IQ/DUT/Rx Beamforming ==
  data_bus_in : Inport
  steering_vector : Inport  Port=2
  capture_src : Inport  Port=3
  mvdr_enable : Inport  Port=4
  diag_loading : Inport  Port=5
  Deinterleave Complex : Subsystem  mask(Deinterleave Complex){}
      mask help: Deinterleave real and imaginary components from input vector. Output is a vector with half the length of the input.
      mask Display: fprintf('Deinterleave\nComplex');
  Input Gate : Subsystem
  Input Scaling : Subsystem
  "Interleave Complex " : Subsystem  mask(Interleave Complex){}
      mask help: Interleave real and imaginary components. Output is a vector with twice the length of the input.
      mask Display: fprintf('Interleave\nComplex');
  MVDR HDL : Subsystem
  Output Selector : Subsystem
  data_bus_out : Outport
  computed_weights : Outport  Port=2
  wires:
  Output Selector/1(data_bus_out) -> data_bus_out/1
  steering_vector/1 -> Deinterleave Complex/1(u)
  MVDR HDL/1(data_bus_out) -> Output Selector/4(mvdr_out_bus)
  data_bus_in/1 -> Output Selector/2(adc_data_bus), Input Scaling/1(data_bus_in)
  MVDR HDL/2(computed_weights) -> "Interleave Complex "/1(u)
  "Interleave Complex "/1(y) -> computed_weights/1
  Deinterleave Complex/1(y) -> MVDR HDL/2(steering_vector)
  mvdr_enable/1 -> Input Gate/1(enable)
  capture_src/1 -> Output Selector/1(src_sel)
  Input Scaling/1(data_bus_out) -> Input Gate/2(data_bus_in)
  Input Gate/1(mvdr_in_bus) -> Output Selector/3(mvdr_in_bus), MVDR HDL/1(data_bus_in)
  diag_loading/1 -> MVDR HDL/3(diag_loading)

== system TxSteering_RxMVDR_4x4_HDL_IQ/DUT/Rx Data Capture ==
  capture_length : Inport
  capture_start : Inport  Port=2
  Bus Element In : Inport  Port=3  PortName=data_bus_in  Element=data
  Bus Element In1 : Inport  Port=3  PortName=data_bus_in  Element=valid
  s2mm_ready : Inport  Port=4
  Delay{,1..2,4} (4 alike) : Delay  DelayLength=1
  Detect Rise Positive : simulink/Logic and Bit Operations/Detect Rise Positive  vinit=0  OutDataTypeStr=boolean
  One-Shot Capture Control : Subsystem
      settings: PortSchema="{\"entries\":[{\"content\":{\"sides\":[{\"content\":{\"connectorIds\":[\"In1\",\"In2\",\"In3\"]},\"type\":\"ConnectorPlacement.EquallySpacedRectSide\",\"uuid\":\"6f09e145-48ee-41d2-bec3-6a733c9106b2\"},{\"content\":{\"connectorIds\":[\"Out1\",\"Out2\",\"In4\"],\"side\":\"RIGHT\"},\"type\":\"ConnectorPlacement.EquallySpacedRectSide\",\"uuid\":\"546a5f38-a809-4883-a76f-61cab94f6d84\"},{\"content\":{\"side\":\"TOP\"},\"type\":\"ConnectorPlacement.EquallySpacedRectSide\",\"uuid\":\"11739b25-d16f-46c4-9eb7-ceb525177655\"}]},\"type\":\"ConnectorPlacement.EquallySpacedConnector\",\"uuid\":\"2379cc98-1392-4372-a564-c1eaf6dbd020\"}],\"packageUris\":[\"http://schema.mathworks.com/mf0/Connector/R2020b\"],\"version\":\"1.0\"}"
  Stream FIFO : Subsystem
      settings: PortSchema="{\"entries\":[{\"content\":{\"sides\":[{\"content\":{\"connectorIds\":[\"In1\",\"In2\",\"In3\",\"Out4\"]},\"type\":\"ConnectorPlacement.EquallySpacedRectSide\",\"uuid\":\"d06c0eab-b8f3-426a-85c0-c3dabc96b0eb\"},{\"content\":{\"connectorIds\":[\"Out1\",\"Out2\",\"Out3\",\"In4\"],\"side\":\"RIGHT\"},\"type\":\"ConnectorPlacement.EquallySpacedRectSide\",\"uuid\":\"fc299245-065a-4284-92f2-e933e11c4572\"},{\"content\":{\"side\":\"TOP\"},\"type\":\"ConnectorPlacement.EquallySpacedRectSide\",\"uuid\":\"8e810d87-ed8e-4951-8437-f6335fefacf7\"}]},\"type\":\"ConnectorPlacement.EquallySpacedConnector\",\"uuid\":\"c15e4701-36e6-4d1a-8e5e-6e8c97e61f22\"}],\"packageUris\":[\"http://schema.mathworks.com/mf0/Connector/R2020b\"],\"version\":\"1.0\"}"
  s2mm_data : Outport  VectorParamsAs1DForOutWhenUnconnected=off
  s2mm_valid : Outport  Port=2  VectorParamsAs1DForOutWhenUnconnected=off
  s2mm_last : Outport  Port=3  VectorParamsAs1DForOutWhenUnconnected=off
  wires:
  capture_length/1 -> Delay2/1
  Bus Element In1/1 -> Delay1/1
  Bus Element In/1 -> Delay/1
  capture_start/1 -> Delay4/1
  Stream FIFO/4(readyOut) -> One-Shot Capture Control/4(readyIn)
  Delay1/1 -> One-Shot Capture Control/1(validIn)
  Delay2/1 -> One-Shot Capture Control/3(length)
  Delay4/1 -> Detect Rise Positive/1
  Detect Rise Positive/1 -> One-Shot Capture Control/2(start)
  Delay/1 -> Stream FIFO/1(dataIn)
  One-Shot Capture Control/1(validOut) -> Stream FIFO/2(validIn)
  Stream FIFO/1(dataOut) -> s2mm_data/1
  Stream FIFO/2(validOut) -> s2mm_valid/1
  s2mm_ready/1 -> Stream FIFO/4(readyIn)
  One-Shot Capture Control/2(lastOut) -> Stream FIFO/3(lastIn)
  Stream FIFO/3(lastOut) -> s2mm_last/1

== system TxSteering_RxMVDR_4x4_HDL_IQ/DUT/Rx Input Preparation ==
  internal_loopback : Inport
  rx_cal_coeffs : Inport  Port=2
  rx_data_bus_in : Inport  Port=3
  tx_data_bus_in : Inport  Port=4
  Apply Calibration Coefficients : Subsystem
  Deinterleave Complex : Subsystem  mask(Deinterleave Complex){}
      mask help: Deinterleave real and imaginary components from input vector. Output is a vector with half the length of the input.
      mask Display: fprintf('Deinterleave\nComplex');
  Delay : Delay  DelayLength=1
  Switch : Switch  Criteria=u2 > Threshold  SaturateOnIntegerOverflow=off  InputSameDT=off
  data_bus_out : Outport  VectorParamsAs1DForOutWhenUnconnected=off
  wires:
  rx_cal_coeffs/1 -> Deinterleave Complex/1(u)
  Delay/1 -> data_bus_out/1
  internal_loopback/1 -> Switch/2
  Switch/1 -> Delay/1
  tx_data_bus_in/1 -> Switch/1
  Deinterleave Complex/1(y) -> Apply Calibration Coefficients/2(coeffIn)
  rx_data_bus_in/1 -> Apply Calibration Coefficients/1(InBus)
  Apply Calibration Coefficients/1(OutBus) -> Switch/3

== system TxSteering_RxMVDR_4x4_HDL_IQ/DUT/To DAC Interface ==
  data_bus_in : Inport
  Complex to Real-Imag : ComplexToRealImag
  Data Type Conversion : DataTypeConversion  OutDataTypeStr=int16  ConvertRealWorld=Stored Integer (SI)  SaturateOnIntegerOverflow=off  RndMeth=Floor
  Delay : Delay  DelayLength=1
  Demux : Demux
  Demux1 : Demux
  From Data Bus : Subsystem  mask(From Data Bus){dummy=0}
      mask help: Convert a streaming Data Bus to individual Data and Valid signals.
      mask Display:
      | port_label('output',1,'data');
      | port_label('output',2,'valid');
  ch1_i_data : Outport
  ch1_q_data : Outport  Port=2
  ch1_valid : Outport  Port=3
  ch2_i_data : Outport  Port=4
  ch2_q_data : Outport  Port=5
  ch2_valid : Outport  Port=6
  ch3_i_data : Outport  Port=7
  ch3_q_data : Outport  Port=8
  ch3_valid : Outport  Port=9
  ch4_i_data : Outport  Port=10
  ch4_q_data : Outport  Port=11
  ch4_valid : Outport  Port=12
  wires:
  data_bus_in/1 -> Delay/1
  From Data Bus/1(data) -> Data Type Conversion/1
  Demux/1 -> ch1_i_data/1
  Demux1/1 -> ch1_q_data/1
  From Data Bus/2(valid) -> ch1_valid/1, ch2_valid/1, ch4_valid/1, ch3_valid/1
  Demux/2 -> ch2_i_data/1
  Demux1/2 -> ch2_q_data/1
  Demux/3 -> ch3_i_data/1
  Demux1/3 -> ch3_q_data/1
  Demux/4 -> ch4_i_data/1
  Demux1/4 -> ch4_q_data/1
  Data Type Conversion/1 -> Complex to Real-Imag/1
  Complex to Real-Imag/1 -> Demux/1
  Complex to Real-Imag/2 -> Demux1/1
  Delay/1 -> From Data Bus/1(bus)

== system TxSteering_RxMVDR_4x4_HDL_IQ/DUT/Tx Signal Generation ==
  nco_enable : Inport
  nco_inc : Inport  Port=2
  gain : Inport  Port=3
  steering_coeffs : Inport  Port=4
  Calibration NCO : Subsystem
  Demux : Demux  Outputs=2
  Generate Steering Channels : Subsystem  TreatAsAtomicUnit=on
  Multiport Switch : MultiPortSwitch  DataPortOrder=Zero-based contiguous  Inputs=2  zeroidx=on  SaturateOnIntegerOverflow=off  InputSameDT=off
  Sum Channels : Subsystem
  To Data Bus : Subsystem  mask(To Data Bus){dummy=0}
      mask help: Create a streaming Data Bus from Data and Valid signals.
      mask Display:
      | port_label('input',1,'data');
      | port_label('input',2,'valid');
  To Data Bus1 : Subsystem  mask(To Data Bus){dummy=0}
      mask help: Create a streaming Data Bus from Data and Valid signals.
      mask Display:
      | port_label('input',1,'data');
      | port_label('input',2,'valid');
  Tx Source LUT : Subsystem
  Tx Sources - Spectrum : SpectrumAnalyzer  NumInputPorts=2  WindowPosition=[967.000000,252.000000,691.000000,497.000000,]  ScopeFrameLocation=window  Method=Welch  SampleRate=245760000  Span=245760000  StartFrequency=-122880000  StopFrequency=122880000  AveragingMethod=Running  YLimits=[-110.04486526,19.60704772]  ShowLegend=on
      settings: OpenAtSimulationStart=off
  data_bus_out : Outport
  wires:
  gain/1 -> Generate Steering Channels/3(gain)
  steering_coeffs/1 -> Generate Steering Channels/4(steering_coeffs)
  Generate Steering Channels/1(data_out) -> Sum Channels/1(data_in)
  Generate Steering Channels/2(valid_out) -> Sum Channels/2(valid_in)
  Tx Source LUT/1(data_out) -> Demux/1, Generate Steering Channels/1(data_in)
  Tx Source LUT/2(valid_out) -> Generate Steering Channels/2(valid_in)
  Sum Channels/2(valid_out) -> To Data Bus/2(valid)
  Sum Channels/1(data_out) -> To Data Bus/1(data)
  Demux/1 -> Tx Sources - Spectrum/1  "Tx Source 1"
  Demux/2 -> Tx Sources - Spectrum/2  "Tx Source 2"
  nco_inc/1 -> Calibration NCO/1(inc)
  Calibration NCO/1(data_out) -> To Data Bus1/1(data)
  Calibration NCO/2(valid_out) -> To Data Bus1/2(valid)
  nco_enable/1 -> Multiport Switch/1
  To Data Bus1/1(bus) -> Multiport Switch/3
  To Data Bus/1(bus) -> Multiport Switch/2
  Multiport Switch/1 -> data_bus_out/1

== system TxSteering_RxMVDR_4x4_HDL_IQ/Loopback Channel/Apply Channel Noise ==
  In1 : Inport
  Add : Sum
  Colored Noise : dspsrcs4/Colored Noise  Color=white  InverseFrequencyPower=1  BoundedOutput=off  NumChannels=4  OutputDataType=double  SamplesPerFrame=1  SampleTime=1/FPGAClkRate  RandomStream=mt19937ar with seed  Seed=67  SimulateUsing=Interpreted execution
  Colored Noise1 : dspsrcs4/Colored Noise  Color=white  InverseFrequencyPower=1  BoundedOutput=off  NumChannels=4  OutputDataType=double  SamplesPerFrame=1  SampleTime=1/FPGAClkRate  RandomStream=mt19937ar with seed  Seed=69  SimulateUsing=Interpreted execution
  Gain : Gain  Gain=5e-3
  Real-Imag to Complex : RealImagToComplex
  Reshape : Reshape
  Rx : Outport
  wires:
  Colored Noise/1 -> Real-Imag to Complex/1
  Gain/1 -> Add/2
  Reshape/1 -> Gain/1
  Colored Noise1/1 -> Real-Imag to Complex/2
  In1/1 -> Add/1
  Real-Imag to Complex/1 -> Reshape/1
  Add/1 -> Rx/1

== system TxSteering_RxMVDR_4x4_HDL_IQ/Loopback Channel/Apply Phase//Amplitude imbalance ==
  In1 : Inport
  Constant : Constant  Value=[1.021*exp(-j*pi/12) 0.967*exp(j*pi/16) 0.945*exp(-j*pi/18) 1.072*exp(j*pi/11) ]  SampleTime=-1
  Product : Product
  Out1 : Outport
  wires:
  Constant/1 -> Product/2
  Product/1 -> Out1/1
  In1/1 -> Product/1

== system TxSteering_RxMVDR_4x4_HDL_IQ/S2MM DMA Behavioral/Unpack to uint32 ==
  dataIn : Inport
  validIn : Inport  Port=2
  Enabled Subsystem : Subsystem  TreatAsAtomicUnit=on
  dataOut : Outport
  validOut : Outport  Port=2
  wires:
  Enabled Subsystem/1(dataOut) -> dataOut/1
  dataIn/1 -> Enabled Subsystem/1(dataIn)
  validIn/1 -> Enabled Subsystem/Enable, validOut/1

== system TxSteering_RxMVDR_4x4_HDL_IQ/Software Interface Behavioral/GenSteeringCoeffs Rx ==
  In1 : Inport
  Constant : Constant  Value=fc  SampleTime=-1
  Constant9 : Constant  Value=0  OutDataTypeStr=double  SampleTime=-1
  Data Type Conversion : DataTypeConversion  OutDataTypeStr=sv_dt  SaturateOnIntegerOverflow=off  RndMeth=Floor
  Interleave Complex 3 : Subsystem  mask(Interleave Complex){}
      mask help: Interleave real and imaginary components. Output is a vector with twice the length of the input.
      mask Display: fprintf('Interleave\nComplex');
  MATLAB System1 : MATLABSystem  System=phased.SteeringVector  PropagationSpeed=physconst( 'LightSpeed' )  IncludeElementResponse=off  NumPhaseShifterBits=0  EnablePolarization=off  SimulateUsing=Interpreted execution  SensorArray=sensorArray
      mask Type: phased.SteeringVector
      mask Display:
      | disp(['Steering' char(10) 'Vector']);
      | port_label('input',1,'Freq');
      | port_label('input',2,'Ang');
  Vector Concatenate : Concatenate  Mode=Multidimensional array
  Out1 : Outport
  wires:
  Vector Concatenate/1 -> MATLAB System1/2
  Constant/1 -> MATLAB System1/1
  In1/1 -> Vector Concatenate/1
  Constant9/1 -> Vector Concatenate/2
  Data Type Conversion/1 -> Interleave Complex 3/1(u)
  MATLAB System1/1 -> Data Type Conversion/1
  Interleave Complex 3/1(y) -> Out1/1

== system TxSteering_RxMVDR_4x4_HDL_IQ/Software Interface Behavioral/GenSteeringCoeffs Tx Source 1 ==
  In1 : Inport
  Constant : Constant  Value=fc  SampleTime=-1
  Constant9 : Constant  Value=0  OutDataTypeStr=double  SampleTime=-1
  Data Type Conversion : DataTypeConversion  OutDataTypeStr=sv_dt  SaturateOnIntegerOverflow=off  RndMeth=Floor
  Interleave Complex 3 : Subsystem  mask(Interleave Complex){}
      mask help: Interleave real and imaginary components. Output is a vector with twice the length of the input.
      mask Display: fprintf('Interleave\nComplex');
  MATLAB System1 : MATLABSystem  System=phased.SteeringVector  PropagationSpeed=physconst( 'LightSpeed' )  IncludeElementResponse=off  NumPhaseShifterBits=0  EnablePolarization=off  SimulateUsing=Interpreted execution  SensorArray=sensorArray
      mask Type: phased.SteeringVector
      mask Display:
      | disp(['Steering' char(10) 'Vector']);
      | port_label('input',1,'Freq');
      | port_label('input',2,'Ang');
  Vector Concatenate : Concatenate  Mode=Multidimensional array
  Out1 : Outport
  wires:
  Constant9/1 -> Vector Concatenate/2
  In1/1 -> Vector Concatenate/1
  Constant/1 -> MATLAB System1/1
  Vector Concatenate/1 -> MATLAB System1/2
  Data Type Conversion/1 -> Interleave Complex 3/1(u)
  MATLAB System1/1 -> Data Type Conversion/1
  Interleave Complex 3/1(y) -> Out1/1

== system TxSteering_RxMVDR_4x4_HDL_IQ/Software Interface Behavioral/GenSteeringCoeffs Tx Source 2 ==
  In1 : Inport
  Constant : Constant  Value=fc  SampleTime=-1
  Constant9 : Constant  Value=0  OutDataTypeStr=double  SampleTime=-1
  Data Type Conversion : DataTypeConversion  OutDataTypeStr=sv_dt  SaturateOnIntegerOverflow=off  RndMeth=Floor
  Interleave Complex 3 : Subsystem  mask(Interleave Complex){}
      mask help: Interleave real and imaginary components. Output is a vector with twice the length of the input.
      mask Display: fprintf('Interleave\nComplex');
  MATLAB System1 : MATLABSystem  System=phased.SteeringVector  PropagationSpeed=physconst( 'LightSpeed' )  IncludeElementResponse=off  NumPhaseShifterBits=0  EnablePolarization=off  SimulateUsing=Interpreted execution  SensorArray=sensorArray
      mask Type: phased.SteeringVector
      mask Display:
      | disp(['Steering' char(10) 'Vector']);
      | port_label('input',1,'Freq');
      | port_label('input',2,'Ang');
  Vector Concatenate : Concatenate  Mode=Multidimensional array
  Out1 : Outport
  wires:
  Vector Concatenate/1 -> MATLAB System1/2
  Constant/1 -> MATLAB System1/1
  In1/1 -> Vector Concatenate/1
  Constant9/1 -> Vector Concatenate/2
  Data Type Conversion/1 -> Interleave Complex 3/1(u)
  MATLAB System1/1 -> Data Type Conversion/1
  Interleave Complex 3/1(y) -> Out1/1

== system TxSteering_RxMVDR_4x4_HDL_IQ/Software Interface Behavioral/Interleave Complex 3 ==
  u : Inport
  interleave_complex_fcn : MATLAB Function  TreatAsAtomicUnit=on
  y : Outport
  wires:
  interleave_complex_fcn/1(y) -> y/1
  u/1 -> interleave_complex_fcn/1(u)

== system TxSteering_RxMVDR_4x4_HDL_IQ/Software Interface Behavioral/Process Beam Data ==
  Data : Inport
  Enable : EnablePort
  AGC : commrfcorlib/AGC  LegacyMode=off  DetectorMethod=Rectifier  LoopMethod=Linear  UpdatePeriod=100  StepSize=0.1  AdaptationStepSize=1e-3  DesiredOutputPower=1  AveragingLength=256  MaximumGain=30  MaxPowerGain=60  GainOutputPort=off  InputPowerOutputPort=off  SimulateUsing=Interpreted execution
  QPSK Receiver : MATLAB Function  TreatAsAtomicUnit=on  mask{infoStruct=testSrc1}
      mask prompts: infoStruct "Source info struct:"
      mask init:
      | FrameLength = infoStruct.FrameLength;
      | SamplesPerSymbol = infoStruct.SamplesPerSymbol;
      | PreambleLength = infoStruct.PreambleLength;
      | mfCoeffs = infoStruct.mfCoeffs;
      | rrcCoeffs = infoStruct.rrcCoeffs;
  Reshape : Reshape  OutputDimensionality=Column vector (2-D)
  Rx Beam - Constellation : ConstellationDiagram  WindowPosition=[2316.000000,299.000000,533.000000,556.000000,]  Visible=on  ScopeFrameLocation=window  XLimits=[-1,1]  YLimits=[-1,1]  DefaultConfigurationName=comm.scopes.ConstellationDiagramBlockCfg
  To Workspace : ToWorkspace  VariableName=sim_beam_data  SampleTime=-1
      settings: Save2DSignal=2-D array (concatenate along first dimension)
  wires:
  Data/1 -> Reshape/1
  Reshape/1 -> QPSK Receiver/1(dataIn), To Workspace/1
  QPSK Receiver/1(dataOut) -> AGC/1
  AGC/1 -> Rx Beam - Constellation/1

== system TxSteering_RxMVDR_4x4_HDL_IQ/DUT/Combine Steering Coeff Regs/Deinterleave Complex ==
  u : Inport
  deinterleave_complex_fcn : MATLAB Function  TreatAsAtomicUnit=on
  y : Outport
  wires:
  deinterleave_complex_fcn/1(y) -> y/1
  u/1 -> deinterleave_complex_fcn/1(u)

== system TxSteering_RxMVDR_4x4_HDL_IQ/DUT/Combine Steering Coeff Regs/Deinterleave Complex1 ==
  u : Inport
  deinterleave_complex_fcn : MATLAB Function  TreatAsAtomicUnit=on
  y : Outport
  wires:
  u/1 -> deinterleave_complex_fcn/1(u)
  deinterleave_complex_fcn/1(y) -> y/1

== system TxSteering_RxMVDR_4x4_HDL_IQ/DUT/From ADC Interface/To Data Bus ==
  data : Inport
  valid : Inport  Port=2
  Bus Creator : BusCreator  Inputs=2
  bus : Outport  VectorParamsAs1DForOutWhenUnconnected=off
  wires:
  Bus Creator/1 -> bus/1
  data/1 -> Bus Creator/1  "data"
  valid/1 -> Bus Creator/2  "valid"

== system TxSteering_RxMVDR_4x4_HDL_IQ/DUT/Rx Beamforming/Deinterleave Complex ==
  u : Inport
  deinterleave_complex_fcn : MATLAB Function  TreatAsAtomicUnit=on
  y : Outport
  wires:
  deinterleave_complex_fcn/1(y) -> y/1
  u/1 -> deinterleave_complex_fcn/1(u)

== system TxSteering_RxMVDR_4x4_HDL_IQ/DUT/Rx Beamforming/Input Gate ==
  enable : Inport
  data_bus_in : Inport  Port=2
  AND : Logic  IconShape=distinctive  AllPortsSameDT=off  OutDataTypeStr=boolean
  From Data Bus : Subsystem  mask(From Data Bus){dummy=0}
      mask help: Convert a streaming Data Bus to individual Data and Valid signals.
      mask Display:
      | port_label('output',1,'data');
      | port_label('output',2,'valid');
  To Data Bus1 : Subsystem  mask(To Data Bus){dummy=0}
      mask help: Create a streaming Data Bus from Data and Valid signals.
      mask Display:
      | port_label('input',1,'data');
      | port_label('input',2,'valid');
  mvdr_in_bus : Outport
  wires:
  data_bus_in/1 -> From Data Bus/1(bus)
  From Data Bus/1(data) -> To Data Bus1/1(data)
  To Data Bus1/1(bus) -> mvdr_in_bus/1
  From Data Bus/2(valid) -> AND/1
  enable/1 -> AND/2
  AND/1 -> To Data Bus1/2(valid)

== system TxSteering_RxMVDR_4x4_HDL_IQ/DUT/Rx Beamforming/Input Scaling ==
  Bus Element In : Inport  PortName=data_bus_in  Element=data
  Bus Element In1 : Inport  PortName=data_bus_in  Element=valid
  Compute Input Magnitude : Subsystem
  Compute Magnitude Inverse Scale : Subsystem
  Data Type Duplicate : DataTypeDuplicate
  Data Type Conversion : DataTypeConversion  RndMeth=Floor
  Delay{1,3..5,7} (5 alike) : Delay  DelayLength=1
  Delay10 : Delay  DelayLength=rx_mag_delay
  Delay11 : Delay  DelayLength=rx_mag_delay
  Delay2 : Delay
  Delay6 : Delay
  Delay8 : Delay  DelayLength=rx_mag_inverse_delay
  Delay9 : Delay  DelayLength=rx_mag_inverse_delay
  Product : Product
  Reshape : Reshape  OutputDimensionality=Row vector (2-D)
  Bus Element Out : Outport  PortName=data_bus_out  Element=data
  Bus Element Out1 : Outport  PortName=data_bus_out  Element=valid
  wires:
  Product/1 -> Delay6/1
  Delay5/1 -> Product/2
  Delay6/1 -> Data Type Conversion/1
  Delay7/1 -> Product/1
  Delay1/1 -> Delay2/1
  Data Type Conversion/1 -> Data Type Duplicate/2, Delay3/1
  Delay3/1 -> Bus Element Out/1
  Delay2/1 -> Delay4/1
  Delay4/1 -> Bus Element Out1/1
  Bus Element In/1 -> Reshape/1
  Bus Element In1/1 -> Delay11/1, Compute Input Magnitude/2(valid_in)
  Compute Input Magnitude/1(mag) -> Compute Magnitude Inverse Scale/1(mag_in)
  Reshape/1 -> Delay10/1, Data Type Duplicate/1, Compute Input Magnitude/1(data_in)
  Compute Magnitude Inverse Scale/1(scale_out) -> Delay5/1
  Compute Input Magnitude/2(mag_valid) -> Compute Magnitude Inverse Scale/2(mag_valid)
  Delay8/1 -> Delay1/1
  Delay9/1 -> Delay7/1
  Delay10/1 -> Delay9/1
  Delay11/1 -> Delay8/1

== system TxSteering_RxMVDR_4x4_HDL_IQ/DUT/Rx Beamforming/Interleave Complex  ==
  u : Inport
  interleave_complex_fcn : MATLAB Function  TreatAsAtomicUnit=on
  y : Outport
  wires:
  u/1 -> interleave_complex_fcn/1(u)
  interleave_complex_fcn/1(y) -> y/1
